simulink model "Sys2019"  (R2019b)
settings: Solver=ode45  StartTime=0.0  StopTime=.5  RelTol=1e-3  EnableMultiTasking=on
PreLoadFcn:
  | CONSTANTS
  | DEFAULT
  | Model
InitFcn:
  | CONSTANTS
  | DEFAULT
  | Model
values from neighbouring files (symbols this model uses):
  Amp0d = [.25 8]    [Model.m]
  Amp0n = [-3.125 -92]    [Model.m]
  Amp1d = [.25 8]    [Model.m]
  Amp1n = [-3.125 -92]    [Model.m]
  AmpSat0 = 24    [Model.m]
  AmpSat1 = 24    [Model.m]
  BackEMF0 = 0.0048    [Model.m]
  BackEMF1 = 0.0048    [Model.m]
  CtlSat0 = 4.5    [Model.m]
  CtlSat1 = 4.5    [Model.m]
  Elec0d = [.0000873 1.13]    [Model.m]
  Elec0n = [0 1]    [Model.m]
  Elec1d = [.0000873 1.13]    [Model.m]
  Elec1n = [0 1]    [Model.m]
  FB0 = 0.9    [Model.m]
  FB1 = 0.9    [Model.m]
  PID0 = [-0.0502 -0.00115 -0.0105]    [Model.m]
  PID1 = [-0.0502 -0.00115 -0.0105]    [Model.m]
  Sens0 = 1.11111    [Model.m]
  Sens1 = 1.11111    [Model.m]
  TConst0 = 0.0047    [Model.m]
  TConst1 = 0.0047    [Model.m]
libraries: simulink x6
settings Model: Creator=Leos  LastModifiedBy=matti
settings DataIOCC: SaveFormat=Array  ReturnWorkspaceOutputs=off
settings OptimizationCC: ExpressionDepthLimit=2147483647  LifeSpan=inf
settings DebuggingCC: AlgebraicLoopMsg=none  UnderspecifiedInitializationDetection=Classic  MergeDetectMultiDrivingBlocksExec=none  SolverPrmCheckMsg=warning  FcnCallInpInsideContextMsg=warning  StateNameClashWarn=warning  SFUnexpectedBacktrackingDiag=warning  SFNoUnconditionalDefaultTransitionDiag=warning  SFExecutionAtInitializationDiag=none  ArithmeticOperatorsInVariantConditions=warning
settings HardwareCC: ProdBitPerPointer=32  ProdBitPerSizeT=32  ProdBitPerPtrDiffT=32  ProdLargestAtomicFloat=None  ProdIntDivRoundTo=Undefined  ProdEndianess=Unspecified  ProdWordSize=32  ProdHWDeviceType=32-bit Generic
settings ModelReferenceCC: PropagateSignalLabelsOutOfModel=off
settings SFSimCC: SimUseLocalCustomCode=off  CustomCodeUndefinedFunction=UseInterfaceOnly
settings RTWCC: RTWUseLocalCustomCode=off
settings CodeAppCC: StateflowObjectComments=on
settings GRTTargetCC: TargetLangStandard=C89/C90 (ANSI)  GeneratePreprocessorConditionals=Disable all  CombineOutputUpdateFcns=off  GRTInterface=on
settings ConfigComp: CovMetricSettings=dw  CovHtmlReporting=on  CovSaveCumulativeToWorkspaceVar=on  CovSaveSingleToWorkspaceVar=on  CovExternalEMLEnable=off  CovSFcnEnable=off

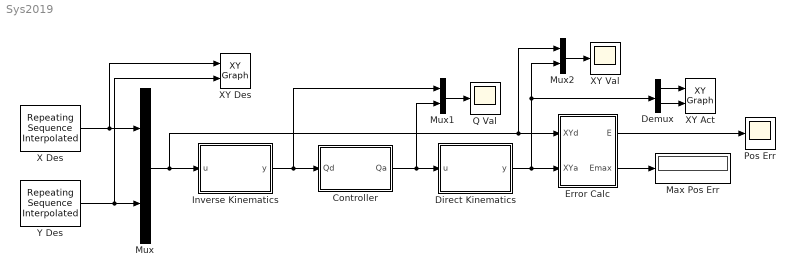
== system Sys2019 ==
  Controller : Subsystem
  Demux : Demux  Outputs=2
  Direct Kinematics : MATLAB Function  TreatAsAtomicUnit=on
  Error Calc : Subsystem
  Inverse Kinematics : MATLAB Function  TreatAsAtomicUnit=on
  Max Pos Err : Display
  Mux : Mux  Inputs=2
  Mux1 : Mux  Inputs=2
  Mux2 : Mux  Inputs=2
  Pos Err : Scope
  Q Val : Scope
  X Des : simulink/Sources/Repeating Sequence Interpolated  OutValues=Xd  TimeValues=Time  LookUpMeth=Interpolation-Use End Values  tsamp=SampleTime  OutMin=[]  OutMax=[]  OutDataTypeStr=double  OutputDataTypeScalingMode=double  OutDataType=fixdt(0,8)  OutScaling=2^-10
  XY Act : simulink/Sinks/XY Graph  xmin=-100  xmax=200  ymin=-100  ymax=200  st=-1
  XY Des : simulink/Sinks/XY Graph  xmin=-100  xmax=200  ymin=-100  ymax=200  st=-1
  XY Val : Scope
  Y Des : simulink/Sources/Repeating Sequence Interpolated  OutValues=Yd  TimeValues=Time  LookUpMeth=Interpolation-Use End Values  tsamp=SampleTime  OutMin=[]  OutMax=[]  OutDataTypeStr=double  OutputDataTypeScalingMode=double  OutDataType=fixdt(0,8)  OutScaling=2^-10
  wires:
  Demux/2 -> XY Act/2
  Direct Kinematics/1(y) -> Mux2/2, Demux/1, Error Calc/2(XYa)
  Demux/1 -> XY Act/1
  Mux/1 -> Inverse Kinematics/1(u), Mux2/1, Error Calc/1(XYd)
  Error Calc/2(Emax) -> Max Pos Err/1
  Error Calc/1(E) -> Pos Err/1
  Inverse Kinematics/1(y) -> Controller/1(Qd), Mux1/1
  Mux1/1 -> Q Val/1
  Mux2/1 -> XY Val/1
  Controller/1(Qa) -> Mux1/2, Direct Kinematics/1(u)
  Y Des/1 -> XY Des/2, Mux/2
  X Des/1 -> XY Des/1, Mux/1

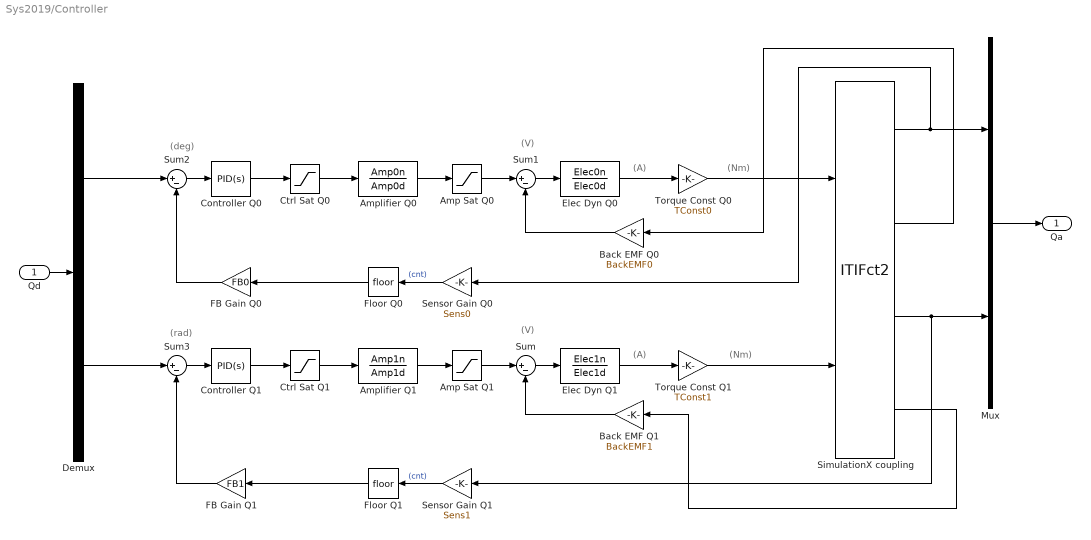
== system Sys2019/Controller ==
  note: (Nm)
  note: (V)
  note: (A)
  note: (A)
  note: (rad)
  note: (deg)
  note: (V)
  note: (Nm)
  Qd : Inport
  Amp Sat Q0 : Saturate  UpperLimit=AmpSat0  LowerLimit=-AmpSat0
  Amp Sat Q1 : Saturate  UpperLimit=AmpSat1  LowerLimit=-AmpSat1
  Amplifier Q0 : TransferFcn  Numerator=Amp0n  Denominator=Amp0d
  Amplifier Q1 : TransferFcn  Numerator=Amp1n  Denominator=Amp1d
  Back EMF Q0 : Gain  Gain=BackEMF0
  Back EMF Q1 : Gain  Gain=BackEMF1
  Controller Q0 : simulink/Continuous/PID Controller  Controller=PID  Form=Parallel  TimeDomain=Continuous-time  SampleTime=-1  IntegratorMethod=Forward Euler  FilterMethod=Forward Euler  ControllerParametersSource=internal  P=PID0(1)  I=PID0(2)  D=PID0(3)  UseFilter=on  N=100  TunerSelectOption=Transfer Function Based (PID Tuner App)  InitialConditionSource=internal  InitialConditionForIntegrator=0  InitialConditionForFilter=0  DifferentiatorICPrevScaledInput=0  ExternalReset=none  TrackingMode=off  Kt=1  LimitOutput=off  UpperSaturationLimit=inf  LowerSaturationLimit=-inf  LinearizeAsGain=on  AntiWindupMode=none  Kb=1  POutMin=[]  POutMax=[]  IOutMin=[]  IOutMax=[]  DOutMin=[]  DOutMax=[]  NOutMin=[]  NOutMax=[]  SumOutMin=[]  SumOutMax=[]  SaturationOutMin=[]  SaturationOutMax=[]  PParamMin=[]  PParamMax=[]  IParamMin=[]  IParamMax=[]  DParamMin=[]  DParamMax=[]  NParamMin=[]  NParamMax=[]  KbParamMin=[]  KbParamMax=[]  KtParamMin=[]  KtParamMax=[]  KbOutMin=[]  KbOutMax=[]  KtOutMin=[]  KtOutMax=[]  IntegratorOutMin=[]  IntegratorOutMax=[]  FilterOutMin=[]  FilterOutMax=[]  SumI1OutMin=[]  SumI1OutMax=[]  SumI2OutMin=[]  SumI2OutMax=[]  SumI3OutMin=[]  SumI3OutMax=[]  SumI4OutMin=[]  SumI4OutMax=[]  SumDOutMin=[]  SumDOutMax=[]  DifferentiatorOutMin=[]  DifferentiatorOutMax=[]  FilterDiffOutCoefMin=[]  FilterDiffOutCoefMax=[]  ReciprocalOutMin=[]  ReciprocalOutMax=[]  SumDenOutMin=[]  SumDenOutMax=[]  SumNumOutMin=[]  SumNumOutMax=[]  DivideOutMin=[]  DivideOutMax=[]  IntegratorContinuousStateAttributes=''  IntegratorStateMustResolveToSignalObject=off  IntegratorRTWStateStorageClass=Auto  FilterContinuousStateAttributes=''  FilterStateMustResolveToSignalObject=off  FilterRTWStateStorageClass=Auto  ParallelPVariant=InternalParameters  IdealPVariant=Disabled  IVariant=InternalParameters  DVariant=InternalParameters  IntegratorVariant=Continuous  SatVariant=Disabled  AWVariant=Passthrough  PCopyVariant=Disabled  TRVariant=Disabled  FdbkBlocksVariant=Forward  IdealPFdbkVariant=Disabled  SatFdbkVariant=Disabled  DerivativeFilterVariant=ContFilter  NVariant=InternalParameters  NCopyVariant=Disabled  FilterICVariant=InternalICsFilter  IntegratorICVariant=InternalICs  ExternalResetVariant=Disabled  TRSumVariant=Passthrough  SumFdbkVariant=Disabled  SumVariant=Sum_PID
  Controller Q1 : simulink/Continuous/PID Controller  Controller=PID  Form=Parallel  TimeDomain=Continuous-time  SampleTime=-1  IntegratorMethod=Forward Euler  FilterMethod=Forward Euler  ControllerParametersSource=internal  P=PID1(1)  I=PID1(2)  D=PID1(3)  UseFilter=on  N=100  TunerSelectOption=Transfer Function Based (PID Tuner App)  InitialConditionSource=internal  InitialConditionForIntegrator=0  InitialConditionForFilter=0  DifferentiatorICPrevScaledInput=0  ExternalReset=none  TrackingMode=off  Kt=1  LimitOutput=off  UpperSaturationLimit=inf  LowerSaturationLimit=-inf  LinearizeAsGain=on  AntiWindupMode=none  Kb=1  POutMin=[]  POutMax=[]  IOutMin=[]  IOutMax=[]  DOutMin=[]  DOutMax=[]  NOutMin=[]  NOutMax=[]  SumOutMin=[]  SumOutMax=[]  SaturationOutMin=[]  SaturationOutMax=[]  PParamMin=[]  PParamMax=[]  IParamMin=[]  IParamMax=[]  DParamMin=[]  DParamMax=[]  NParamMin=[]  NParamMax=[]  KbParamMin=[]  KbParamMax=[]  KtParamMin=[]  KtParamMax=[]  KbOutMin=[]  KbOutMax=[]  KtOutMin=[]  KtOutMax=[]  IntegratorOutMin=[]  IntegratorOutMax=[]  FilterOutMin=[]  FilterOutMax=[]  SumI1OutMin=[]  SumI1OutMax=[]  SumI2OutMin=[]  SumI2OutMax=[]  SumI3OutMin=[]  SumI3OutMax=[]  SumI4OutMin=[]  SumI4OutMax=[]  SumDOutMin=[]  SumDOutMax=[]  DifferentiatorOutMin=[]  DifferentiatorOutMax=[]  FilterDiffOutCoefMin=[]  FilterDiffOutCoefMax=[]  ReciprocalOutMin=[]  ReciprocalOutMax=[]  SumDenOutMin=[]  SumDenOutMax=[]  SumNumOutMin=[]  SumNumOutMax=[]  DivideOutMin=[]  DivideOutMax=[]  IntegratorContinuousStateAttributes=''  IntegratorStateMustResolveToSignalObject=off  IntegratorRTWStateStorageClass=Auto  FilterContinuousStateAttributes=''  FilterStateMustResolveToSignalObject=off  FilterRTWStateStorageClass=Auto  ParallelPVariant=InternalParameters  IdealPVariant=Disabled  IVariant=InternalParameters  DVariant=InternalParameters  IntegratorVariant=Continuous  SatVariant=Disabled  AWVariant=Passthrough  PCopyVariant=Disabled  TRVariant=Disabled  FdbkBlocksVariant=Forward  IdealPFdbkVariant=Disabled  SatFdbkVariant=Disabled  DerivativeFilterVariant=ContFilter  NVariant=InternalParameters  NCopyVariant=Disabled  FilterICVariant=InternalICsFilter  IntegratorICVariant=InternalICs  ExternalResetVariant=Disabled  TRSumVariant=Passthrough  SumFdbkVariant=Disabled  SumVariant=Sum_PID
  Ctrl Sat Q0 : Saturate  UpperLimit=CtlSat0  LowerLimit=-CtlSat0
  Ctrl Sat Q1 : Saturate  UpperLimit=CtlSat1  LowerLimit=-CtlSat1
  Demux : Demux  Outputs=2
  Elec Dyn Q0 : TransferFcn  Numerator=Elec0n  Denominator=Elec0d
  Elec Dyn Q1 : TransferFcn  Numerator=Elec1n  Denominator=Elec1d
  FB Gain Q0 : Gain  Gain=FB0
  FB Gain Q1 : Gain  Gain=FB1
  Floor Q0 : Rounding
  Floor Q1 : Rounding
  Mux : Mux  Inputs=2
  Sensor Gain Q0 : Gain  Gain=Sens0
  Sensor Gain Q1 : Gain  Gain=Sens1
  SimulationX coupling : S-Function  FunctionName=ITIFct2  Parameters=ip, port, ts, nIn, nOut  SFunctionDeploymentMode=off  EnableBusSupport=off  mask{ip='localhost', port=4097, ts=0.001, nIn=2, nOut=4}
      mask prompts: ip "Address: ip"; port "Port Number: port [-]"; ts "Communication Step Size: ts [s]"; nIn "Input Vector Dimension (to SimulationX): nIn [-]"; nOut "Output Vector Dimension (from SimulationX): nOut [-]"
      mask help: Coupling Element
  Sum{,1..3} (4 alike) : Sum  Inputs=|+-
  Torque Const Q0 : Gain  Gain=TConst0
  Torque Const Q1 : Gain  Gain=TConst1
  Qa : Outport
  wires:
  Back EMF Q0/1 -> Sum1/2
  Torque Const Q1/1 -> SimulationX coupling/2
  Back EMF Q1/1 -> Sum/2
  FB Gain Q1/1 -> Sum3/2
  Ctrl Sat Q1/1 -> Amplifier Q1/1
  Amp Sat Q0/1 -> Sum1/1
  Controller Q1/1 -> Ctrl Sat Q1/1
  Sum1/1 -> Elec Dyn Q0/1
  SimulationX coupling/1 -> Sensor Gain Q0/1, Mux/1
  Torque Const Q0/1 -> SimulationX coupling/1
  Controller Q0/1 -> Ctrl Sat Q0/1
  Floor Q0/1 -> FB Gain Q0/1
  Amp Sat Q1/1 -> Sum/1
  SimulationX coupling/3 -> Sensor Gain Q1/1, Mux/2
  Floor Q1/1 -> FB Gain Q1/1
  Elec Dyn Q0/1 -> Torque Const Q0/1
  Sensor Gain Q1/1 -> Floor Q1/1  "(cnt)"
  Elec Dyn Q1/1 -> Torque Const Q1/1
  SimulationX coupling/2 -> Back EMF Q0/1
  Sum2/1 -> Controller Q0/1
  Qd/1 -> Demux/1
  Mux/1 -> Qa/1
  Amplifier Q1/1 -> Amp Sat Q1/1
  Sum3/1 -> Controller Q1/1
  SimulationX coupling/4 -> Back EMF Q1/1
  Sensor Gain Q0/1 -> Floor Q0/1  "(cnt)"
  Ctrl Sat Q0/1 -> Amplifier Q0/1
  Amplifier Q0/1 -> Amp Sat Q0/1
  Sum/1 -> Elec Dyn Q1/1
  FB Gain Q0/1 -> Sum2/2
  Demux/1 -> Sum2/1
  Demux/2 -> Sum3/1

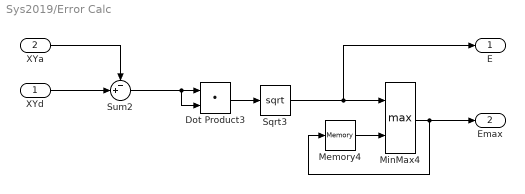
== system Sys2019/Error Calc ==
  XYd : Inport
  XYa : Inport  Port=2
  Dot Product3 : DotProduct  InputSameDT=on  OutDataTypeStr=Inherit: Inherit via internal rule
  Memory4 : Memory
  MinMax4 : MinMax  Function=max  Inputs=2
  Sqrt3 : Sqrt  SaturateOnIntegerOverflow=on
  Sum2 : Sum  Inputs=-+|
  E : Outport
  Emax : Outport  Port=2
  wires:
  XYa/1 -> Sum2/1
  Memory4/1 -> MinMax4/2
  MinMax4/1 -> Emax/1, Memory4/1
  XYd/1 -> Sum2/2
  Sum2/1 -> Dot Product3/2, Dot Product3/1
  Dot Product3/1 -> Sqrt3/1
  Sqrt3/1 -> E/1, MinMax4/1

== matlab function Sys2019/Direct Kinematics ==
  data: u input; y output
function y = DirKin(u)

% This assumes first param is theta_0 and second is theta_1
% COnvert back from gear ratio
theta_0 = u(1) / (-3);
theta_1 = u(2) / (-3);

xpos = 100 * (cosd(theta_0) + cosd(theta_1));
ypos = 100 * (sind(theta_0) + sind(theta_1));

% Return Default Result
y = [ xpos; ypos ];

== matlab function Sys2019/Inverse Kinematics ==
  data: u input; y output
function y = InvKin(u)

% Convert to m from mm
x0 = u(1);
y0 = u(2);

% Compute internal max length
r = sqrt(x0^2 + y0^2);
L = 100;

% Compute intermediate angles of isosceles triangle approximation
phi_1 = acos( (r^2) / (2*L*r) );
phi_2 = angle((x0 + y0*i));
phi_3 = acos( (2*L^2 - r^2) / (2*L^2) );

% Compute final angle of joints
theta_0 = phi_1 + phi_2;
theta_2 = pi - phi_3;
theta_1 = theta_0 - theta_2;

% Convert to degress and account for gear ratio
% Return Default Result
y = (-3) * [ theta_0  * (180/pi); theta_1  * (180/pi)];
